simulink model "inv_switch1"  (Simulink 4.00)
settings: Solver=ode45  StartTime=0.0  StopTime=20e-3  RelTol=1e-3
values from neighbouring files (symbols this model uses):
  C = 500e-6    (= 0.0005)    [inv_switch_1.m]    (also in mehrw_1.m = eye(10,10); mehrw_2.m = eye(10,10); mehrw_3.m = eye(10,10); mehrw_4.m = eye(10,10))
  L = 0.5e-3    (= 0.0005)    [inv_switch_1.m]
  Rp = 1    [inv_switch_1.m]
libraries: simulink3 x1
settings Model: LastModifiedBy=Administrator  MaxDataPoints=200  BlockReductionOpt=off

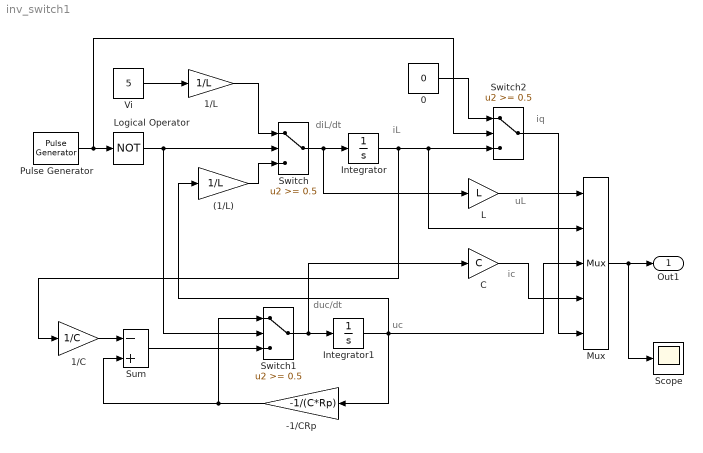
== system inv_switch1 ==
  note: uc
  note: duc/dt
  note: diL/dt
  note: iL
  note: uL
  note: ic
  note: iq
  (1/L) : Gain  Gain=1/L  Multiplication=Element-wise(K.*u)  SaturateOnIntegerOverflow=on
  -1/CRp : Gain  Orientation=left  Gain=-1/(C*Rp)  Multiplication=Element-wise(K.*u)  SaturateOnIntegerOverflow=on
  0 : Constant  Value=0
  1/C : Gain  Gain=1/C  Multiplication=Element-wise(K.*u)  SaturateOnIntegerOverflow=on
  1/L : Gain  Gain=1/L  Multiplication=Element-wise(K.*u)  SaturateOnIntegerOverflow=on
  C : Gain  Gain=C  Multiplication=Element-wise(K.*u)  SaturateOnIntegerOverflow=on
  Integrator : Integrator  ExternalReset=none  InitialConditionSource=internal  InitialCondition=0  LimitOutput=off  UpperSaturationLimit=inf  LowerSaturationLimit=-inf  ShowSaturationPort=off  ShowStatePort=off  AbsoluteTolerance=auto
  Integrator1 : Integrator  ExternalReset=none  InitialConditionSource=internal  InitialCondition=0  LimitOutput=off  UpperSaturationLimit=inf  LowerSaturationLimit=-inf  ShowSaturationPort=off  ShowStatePort=off  AbsoluteTolerance=auto
  L : Gain  Gain=L  Multiplication=Element-wise(K.*u)  SaturateOnIntegerOverflow=on
  Logical Operator : Logic  Operator=NOT  Inputs=2
  Mux : Mux  Inputs=5
      settings: DisplayOption=none
  Pulse Generator : simulink3/Sources/Pulse Generator  period=1/50000  duty=tast  amplitude=1  start=0
  Scope : Scope
      settings: TimeRange=auto  YMin=-5  YMax=5  SaveToWorkspace=off  SaveName=ScopeData  LimitDataPoints=on  MaxDataPoints=5000
  Sum : Sum  Inputs=-+  SaturateOnIntegerOverflow=on
  Switch : Switch  Threshold=0.5
  Switch1 : Switch  Threshold=0.5
  Switch2 : Switch  Threshold=0.5
  Vi : Constant  Value=5
  Out1 : Outport  Port=1
  wires:
  Pulse Generator/1 -> Logical Operator/1, Switch2/2
  1/L/1 -> Switch/1
  Vi/1 -> 1/L/1
  Logical Operator/1 -> Switch/2, Switch1/2
  (1/L)/1 -> Switch/3
  Switch1/1 -> Integrator1/1, C/1
  Switch/1 -> Integrator/1, L/1
  Integrator1/1 -> (1/L)/1, -1/CRp/1, Mux/3
  -1/CRp/1 -> Switch1/1, Sum/2
  Sum/1 -> Switch1/3
  1/C/1 -> Sum/1
  Integrator/1 -> 1/C/1, Switch2/3, Mux/2
  0/1 -> Switch2/1
  Switch2/1 -> Mux/5
  L/1 -> Mux/1
  C/1 -> Mux/4
  Mux/1 -> Out1/1, Scope/1
